simulink model "speed_observer"  (R2023b)
settings: Solver=FixedStepAuto  StartTime=0.0  StopTime=10.0  FixedStep=0.001  RelTol=1e-3
libraries: simulink x5, dsparch4 x3
settings Model: Creator=XHServer  LastModifiedBy=XHServer
settings OptimizationCC: DefaultParameterBehavior=Inlined  UseDivisionForNetSlopeComputation=on  GainParamInheritBuiltInType=on  UseFloatMulNetSlope=on  InlineInvariantSignals=on  EnhancedBackFolding=on  PassReuseOutputArgsAs=Individual arguments  ZeroExternalMemoryAtStartup=off  ZeroInternalMemoryAtStartup=off  EfficientFloat2IntCast=on  OptimizeBlockOrder=speed  DifferentSizesBufferReuse=on  OptimizationCustomize=off  EfficientTunableParamExpr=on
settings DebuggingCC: ParameterTunabilityLossMsg=error
settings SFSimCC: MATLABDynamicMemAlloc=off
settings RTWCC: Description=Create Visual C/C++ Solution File for Embedded Coder  SystemTargetFile=ert.tlc  TemplateMakefile=RTW.MSVCBuild  GenerateReport=on  BuildConfiguration=Faster Runs  LaunchReport=on  RTWCompilerOptimization=on
settings CodeAppCC: ForceParamTrailComments=on  IgnoreCustomStorageClasses=off  OperatorAnnotations=on  SimulinkDataObjDesc=on  SFDataObjDesc=on  InsertBlockDesc=on
settings ERTTargetCC: TargetLangStandard=C99 (ISO)  GenerateSampleERTMain=on  InlinedParameterPlacement=NonHierarchical  ERTCustomFileTemplate=example_file_process.tlc

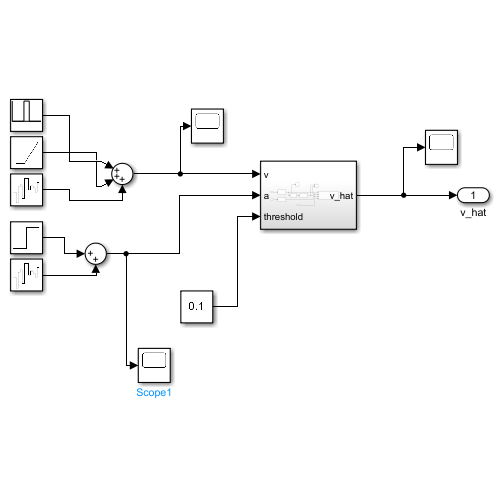
[thumbnail: Simulink's stored preview of the top-level diagram]
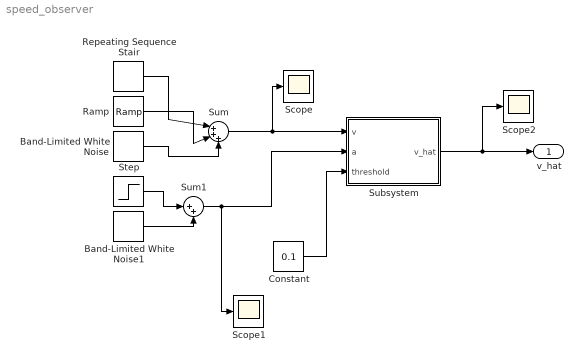
== system speed_observer ==
  Band-Limited White Noise : simulink/Sources/Band-Limited White Noise  Cov=[3e-9]  Ts=0.001  seed=[23341]
  Band-Limited White Noise1 : simulink/Sources/Band-Limited White Noise  Cov=[1e-6]  Ts=0.001  seed=[23341]
  Constant : Constant  Value=0.1
  Ramp : simulink/Sources/Ramp  slope=1  start=1  InitialOutput=0
  Repeating Sequence Stair : simulink/Sources/Repeating Sequence Stair  OutValues=[0 0 1 0 0].'  tsamp=2  OutMin=[]  OutMax=[]  OutDataTypeStr=double  OutputDataTypeScalingMode=double  OutDataType=fixdt(0,8)  ConRadixGroup=Best Precision: Vector-wise  OutScaling=2^-12
  Scope : Scope
  Scope1 : Scope
  Scope2 : Scope
  Step : Step  SampleTime=0
  Subsystem : Subsystem
  Sum : Sum  Inputs=|+++
  Sum1 : Sum  Inputs=|++
  v_hat : Outport  OutDataTypeStr=double  Unit=m/s
  wires:
  Subsystem/1(v_hat) -> Scope2/1, v_hat/1
  Constant/1 -> Subsystem/3(threshold)
  Ramp/1 -> Sum/2
  Repeating Sequence Stair/1 -> Sum/1
  Band-Limited White Noise/1 -> Sum/3
  Sum/1 -> Scope/1, Subsystem/1(v)
  Sum1/1 -> Scope1/1, Subsystem/2(a)
  Step/1 -> Sum1/1
  Band-Limited White Noise1/1 -> Sum1/2

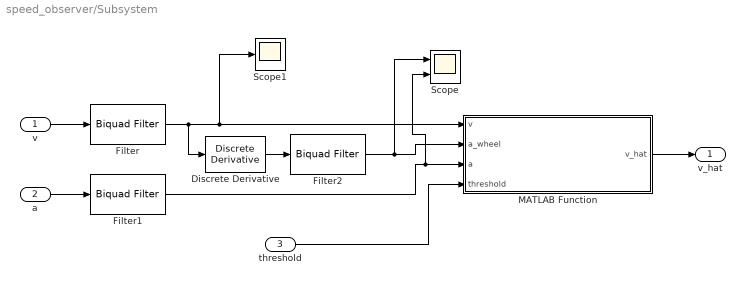
== system speed_observer/Subsystem ==
  v : Inport  OutDataTypeStr=double  Unit=m/s
  a : Inport  Port=2  OutDataTypeStr=double  Unit=m/s^2
  threshold : Inport  Port=3
  Discrete Derivative : simulink/Discrete/Discrete Derivative  gainval=1.0  ICPrevScaledInput=0.0  OutMin=[]  OutMax=[]  OutDataType=fixdt(1, 16)  OutScaling=2^-10  DoSatur=off
  Filter : dsparch4/Biquad Filter  Tag=BlockMethodSubSystem  FilterSource=Dialog parameters  CoeffSource=Specify via dialog  FilterObject=BQF  IIRFiltStruct=Direct form II  BiQuadCoeffs=[1 2 1 1 -1.7347257688092752 0.766006600943263893]  ScaleValues=[0.0078202080334971915;1]  IC=0  ICnum=0  ICden=0  a0Flag=Warning  optimizeScaleValues=on  ScaleValueMode=Specify via input port (g)  InputProcessing=Columns as channels (frame based)  roundingMode=Floor  overflowMode=off  scaleValueFracLength=14  denProdOutputFracLength=30  denAccumFracLength=30  secondMemoryFracLength=15
  Filter1 : dsparch4/Biquad Filter  Tag=BlockMethodSubSystem  FilterSource=Dialog parameters  CoeffSource=Specify via dialog  FilterObject=BQF  IIRFiltStruct=Direct form II  BiQuadCoeffs=[1 2 1 1 -1.7347257688092752 0.766006600943263893]  ScaleValues=[0.0078202080334971915;1]  IC=0  ICnum=0  ICden=0  a0Flag=Warning  optimizeScaleValues=on  ScaleValueMode=Specify via input port (g)  InputProcessing=Columns as channels (frame based)  roundingMode=Floor  overflowMode=off  scaleValueFracLength=14  denProdOutputFracLength=30  denAccumFracLength=30  secondMemoryFracLength=15
  Filter2 : dsparch4/Biquad Filter  Tag=BlockMethodSubSystem  FilterSource=Dialog parameters  CoeffSource=Specify via dialog  FilterObject=BQF  IIRFiltStruct=Direct form II  BiQuadCoeffs=[1 2 1 1 -1.7347257688092752 0.766006600943263893]  ScaleValues=[0.0078202080334971915;1]  IC=0  ICnum=0  ICden=0  a0Flag=Warning  optimizeScaleValues=on  ScaleValueMode=Specify via input port (g)  InputProcessing=Columns as channels (frame based)  roundingMode=Floor  overflowMode=off  scaleValueFracLength=14  denProdOutputFracLength=30  denAccumFracLength=30  secondMemoryFracLength=15
  MATLAB Function : MATLAB Function  TreatAsAtomicUnit=on
  Scope : Scope  NumInputPorts=2
  Scope1 : Scope
  v_hat : Outport  OutDataTypeStr=double  Unit=m/s
  wires:
  MATLAB Function/1(v_hat) -> v_hat/1
  Filter/1 -> Scope1/1, MATLAB Function/1(v), Discrete Derivative/1
  threshold/1 -> MATLAB Function/4(threshold)
  a/1 -> Filter1/1
  v/1 -> Filter/1
  Filter1/1 -> Scope/2, MATLAB Function/3(a)
  Discrete Derivative/1 -> Filter2/1
  Filter2/1 -> Scope/1, MATLAB Function/2(a_wheel)

== matlab function speed_observer/Subsystem/MATLAB Function ==
  data: v input; a_wheel input; v_hat output; a input; threshold input
function v_hat = speed_observer(v,a_wheel,a,threshold)
t=0.001;
% 速度估计，采用阈值切换的办法
% 轮加速度比加速度计高于阈值则切换成加速度计积分
persistent v_storage 
if isempty(v_storage)
   v_storage = 0;
end 
if(a_wheel-a>threshold)%此处仅考虑加速情况
    if(v_storage==0)
        v_storage=v;
    end
    v_hat=v_storage+a*t;
else
    v_hat=v;
    v_storage=0;
end
end
